simulink model "Kittyslx"  (R2022a)
settings: Solver=VariableStepAuto  StartTime=0.0  StopTime=500  RelTol=1e-3
libraries: simulink x1
settings Model: Creator=User  LastModifiedBy=User

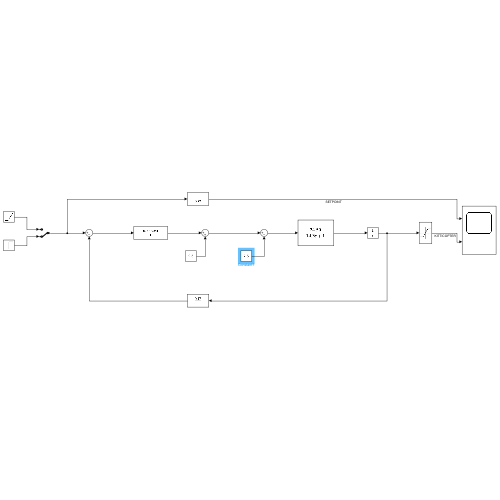
[thumbnail: Simulink's stored preview of the top-level diagram]
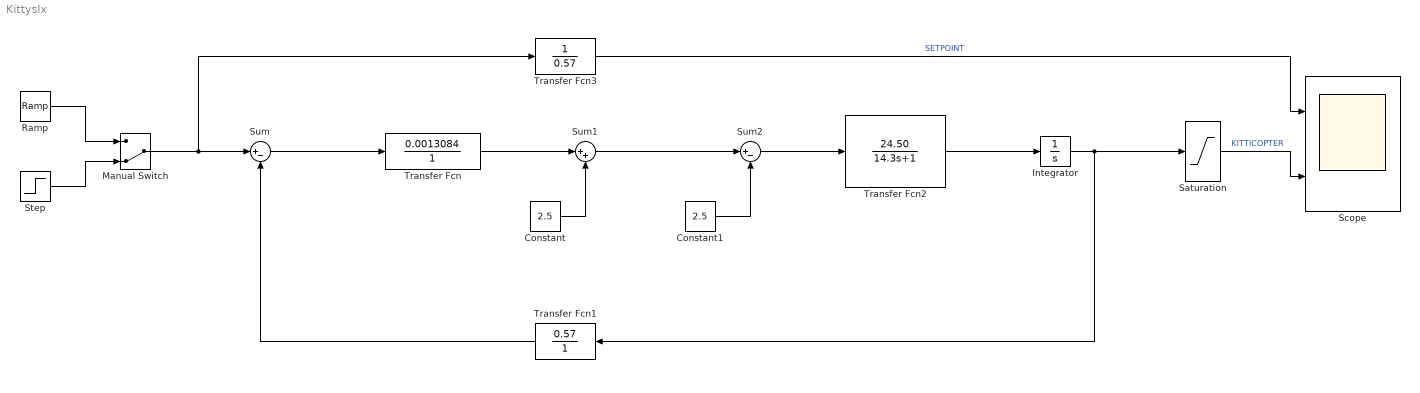
== system Kittyslx ==
  Constant : Constant  Value=2.5
  Constant1 : Constant  Value=2.5
  Integrator : Integrator
  Manual Switch : ManualSwitch  CurrentSetting=0
  Ramp : simulink/Sources/Ramp  slope=1  start=1  InitialOutput=0
  Saturation : Saturate  UpperLimit=3000  LowerLimit=0
  Scope : Scope  NumInputPorts=2
  Step : Step  Time=-0  After=0.57  SampleTime=0
  Sum : Sum  Inputs=|+-
  Sum1 : Sum  Inputs=|++
  Sum2 : Sum  Inputs=|+-
  Transfer Fcn : TransferFcn  Numerator=[0.0013084]  Denominator=[1]
  Transfer Fcn1 : TransferFcn  Numerator=[0.57]  Denominator=[1]
  Transfer Fcn2 : TransferFcn  Numerator=[24.50]  Denominator=[14.3 1]
  Transfer Fcn3 : TransferFcn  Denominator=[0.57]
  wires:
  Manual Switch/1 -> Transfer Fcn3/1, Sum/1
  Sum/1 -> Transfer Fcn/1
  Transfer Fcn/1 -> Sum1/1
  Constant/1 -> Sum1/2
  Sum1/1 -> Sum2/1
  Constant1/1 -> Sum2/2
  Transfer Fcn1/1 -> Sum/2
  Step/1 -> Manual Switch/2
  Sum2/1 -> Transfer Fcn2/1
  Transfer Fcn2/1 -> Integrator/1
  Integrator/1 -> Saturation/1, Transfer Fcn1/1
  Saturation/1 -> Scope/2  "KITTICOPTER"
  Transfer Fcn3/1 -> Scope/1  "SETPOINT"
  Ramp/1 -> Manual Switch/1
